simulink library "euler_equations"  (R2020b)
settings: Solver=VariableStepAuto  StartTime=0.0  StopTime=10.0  RelTol=1e-3
values from neighbouring files (symbols this model uses):
  inv_J = inv(J)    [initial_conditions.m]
  J = diag([Jx Jy Jz])    [initial_conditions.m]
  w0 = [wx0 wy0 wz0]    [initial_conditions.m]
libraries: vrlib x1
settings Model: Creator=whitehole  LastModifiedBy=whitehole

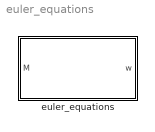
== system euler_equations ==
  euler_equations : Subsystem

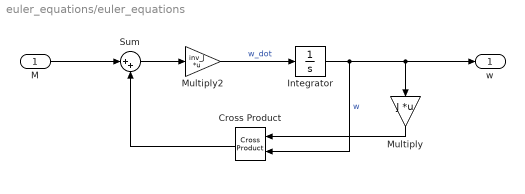
== system euler_equations/euler_equations ==
  M : Inport
  Cross Product : vrlib/Utilities/Cross Product
  Integrator : Integrator  InitialCondition=w0
  Multiply : Gain  Gain=J  Multiplication=Matrix(K*u)
  Multiply2 : Gain  Gain=inv_J  Multiplication=Matrix(K*u)
  Sum : Sum  Inputs=|++
  w : Outport
  wires:
  Integrator/1 -> w/1, Multiply/1, Cross Product/2  "w"
  Sum/1 -> Multiply2/1
  M/1 -> Sum/1
  Multiply2/1 -> Integrator/1  "w_dot"
  Cross Product/1 -> Sum/2
  Multiply/1 -> Cross Product/1
